simulink model "aerotest"  (R2021b)
settings: Solver=VariableStepAuto  StartTime=0.0  StopTime=10.0  RelTol=1e-3
undefined symbols (not defined in the file or in its folder): admireDB
libraries: simulink_extras x103, simulink x24, aerolibatmos2 x1
(part 7 of 13)

== system aerotest/YawMomentCoefficient/MachRegion2/Cymdna ==
  in_bus : Inport
  Bus Selector : BusSelector  OutputSignals=AeroIn_Bus.dNE,AeroIn_Bus.angleOfAttack_deg,AeroIn_Bus.tflow,AeroIn_Bus.tfhigh,AeroIn_Bus.dNA
  Cymdna_ : Subsystem
  Cymdna : Outport
  wires:
  Bus Selector/2 -> Cymdna_/2(angleOfAttack_deg)  "<angleOfAttack_deg>"
  Bus Selector/1 -> Cymdna_/1(dNE)  "<dNE>"
  Bus Selector/3 -> Cymdna_/3(tflow)  "<tflow>"
  Bus Selector/4 -> Cymdna_/4(tfhigh)  "<tfhigh>"
  Bus Selector/5 -> Cymdna_/5(dNA)  "<dNA>"
  in_bus/1 -> Bus Selector/1  "in_bus"
  Cymdna_/1(Cymdna) -> Cymdna/1

== system aerotest/YawMomentCoefficient/MachRegion2/Cymdr ==
  in_bus : Inport
  Bus Selector : BusSelector  OutputSignals=AeroIn_Bus.angleOfAttack_deg,AeroIn_Bus.rud_deg,AeroIn_Bus.angleOfSideslip_deg,AeroIn_Bus.tflow,AeroIn_Bus.tfhigh,AeroIn_Bus.qacorr,AeroIn_Bus.mach_nd
  Cymdr_ : Subsystem
  Cymdr : Outport
  wires:
  Bus Selector/1 -> Cymdr_/1(angleOfAttack_deg)  "<angleOfAttack_deg>"
  Bus Selector/2 -> Cymdr_/2(dR)  "<rud_deg>"
  Bus Selector/3 -> Cymdr_/3(angleOfSideslip_deg)  "<angleOfSideslip_deg>"
  Bus Selector/4 -> Cymdr_/4(tfhigh)  "<tflow>"
  Bus Selector/5 -> Cymdr_/5(tflow)  "<tfhigh>"
  Bus Selector/6 -> Cymdr_/6(qacorr)  "<qacorr>"
  Bus Selector/7 -> Cymdr_/7(mach_nd)  "<mach_nd>"
  in_bus/1 -> Bus Selector/1  "in_bus"
  Cymdr_/1(Cymdr) -> Cymdr/1

== system aerotest/YawMomentCoefficient/MachRegion2/Cymp ==
  in_bus : Inport
  Bus Selector : BusSelector  OutputSignals=AeroIn_Bus.dN,AeroIn_Bus.angleOfAttack_deg,AeroIn_Bus.tflow,AeroIn_Bus.tfhigh,AeroIn_Bus.pc,AeroIn_Bus.qacorr,AeroIn_Bus.mach_nd
  Cymp_ : Subsystem
  Cymp : Outport
  wires:
  Bus Selector/1 -> Cymp_/1(dN)  "<dN>"
  Bus Selector/2 -> Cymp_/2(angleOfAttack_deg)  "<angleOfAttack_deg>"
  Bus Selector/7 -> Cymp_/7(mach_nd)  "<mach_nd>"
  Bus Selector/3 -> Cymp_/3(tflow)  "<tflow>"
  Bus Selector/6 -> Cymp_/6(qacorr)  "<qacorr>"
  Bus Selector/4 -> Cymp_/4(tfhigh)  "<tfhigh>"
  Bus Selector/5 -> Cymp_/5(pc)  "<pc>"
  in_bus/1 -> Bus Selector/1  "in_bus"
  Cymp_/1(Cymp) -> Cymp/1

== system aerotest/YawMomentCoefficient/MachRegion2/Cympbeta ==
  in_bus : Inport
  Bus Selector : BusSelector  OutputSignals=AeroIn_Bus.angleOfSideslip_deg,AeroIn_Bus.angleOfAttack_deg,AeroIn_Bus.pc,AeroIn_Bus.tflow
  Cympbeta_ : Subsystem
  Cympbeta : Outport
  wires:
  Bus Selector/1 -> Cympbeta_/1(angleOfSideslip_deg)  "<angleOfSideslip_deg>"
  Bus Selector/2 -> Cympbeta_/2(angleOfAttack_deg)  "<angleOfAttack_deg>"
  Bus Selector/3 -> Cympbeta_/3(pc)  "<pc>"
  Bus Selector/4 -> Cympbeta_/4(tflow)  "<tflow>"
  Cympbeta_/1(Cympbeta) -> Cympbeta/1
  in_bus/1 -> Bus Selector/1  "in_bus"

== system aerotest/YawMomentCoefficient/MachRegion2/Cymr ==
  in_bus : Inport
  Bus Selector : BusSelector  OutputSignals=AeroIn_Bus.dN,AeroIn_Bus.angleOfAttack_deg,AeroIn_Bus.tflow,AeroIn_Bus.tfhigh,AeroIn_Bus.rc,AeroIn_Bus.mach_nd,AeroIn_Bus.qacorr
  Cymr_ : Subsystem
  Cymr : Outport
  wires:
  Bus Selector/7 -> Cymr_/7(qacorr)  "<qacorr>"
  Bus Selector/6 -> Cymr_/6(mach_nd)  "<mach_nd>"
  Bus Selector/5 -> Cymr_/5(rc)  "<rc>"
  Bus Selector/4 -> Cymr_/4(tfhigh)  "<tfhigh>"
  Bus Selector/3 -> Cymr_/3(tflow)  "<tflow>"
  Bus Selector/2 -> Cymr_/2(angleOfAttack_deg)  "<angleOfAttack_deg>"
  Bus Selector/1 -> Cymr_/1(dN)  "<dN>"
  in_bus/1 -> Bus Selector/1  "in_bus"
  Cymr_/1(Cymr) -> Cymr/1

== system aerotest/YawMomentCoefficient/MachRegion2/Cymrbeta ==
  in_bus : Inport
  Bus Selector : BusSelector  OutputSignals=AeroIn_Bus.angleOfSideslip_deg,AeroIn_Bus.angleOfAttack_deg,AeroIn_Bus.rc,AeroIn_Bus.tflow
  Cymrbeta_ : Subsystem
  Cymrbeta : Outport
  wires:
  Bus Selector/1 -> Cymrbeta_/1(angleOfSideslip_deg)  "<angleOfSideslip_deg>"
  Bus Selector/2 -> Cymrbeta_/2(angleOfAttack_deg)  "<angleOfAttack_deg>"
  Bus Selector/3 -> Cymrbeta_/3(rc)  "<rc>"
  Bus Selector/4 -> Cymrbeta_/4(tflow)  "<tflow>"
  Cymrbeta_/1(Cymrbeta) -> Cymrbeta/1
  in_bus/1 -> Bus Selector/1  "in_bus"

== system aerotest/YawMomentCoefficient/MachRegion2/eoeff ==
  AeroIn_Bus : Inport
  Bus Selector : BusSelector  OutputSignals=mach_nd
  CYMDAYOD_M : Lookup_n-D  NumberOfTableDimensions=1  BreakpointsForDimension1=admireDB.aerodata_asym_ext.CYMDAYOD.breakpoints.M  BreakpointsForDimension3=[5, 7]  Table=admireDB.aerodata_asym_ext.CYMDAYOD.newTable  ExtrapMethod=Clip  InternalRulePriority=Speed  RndMeth=Simplest  InputSameDT=on
  Constant : Constant
  Sum : Sum  Inputs=-+|
  eoeff : Outport
  eieff : Outport  Port=2
  wires:
  Sum/1 -> eieff/1
  CYMDAYOD_M/1 -> eoeff/1, Sum/1
  Constant/1 -> Sum/2
  Bus Selector/1 -> CYMDAYOD_M/1  "<mach_nd>"
  AeroIn_Bus/1 -> Bus Selector/1

== system aerotest/YawMomentCoefficient/MachRegion3/Cymbasic ==
  Constant : Constant  Value=0
  Cymbasic : Outport
  wires:
  Constant/1 -> Cymbasic/1

== system aerotest/YawMomentCoefficient/MachRegion3/Cymbcai ==
  in_bus : Inport
  Bus Selector : BusSelector  OutputSignals=AeroIn_Bus.cai,AeroIn_Bus.angleOfAttack_deg,AeroIn_Bus.angleOfSideslip_deg
  Cymbcai_ : Subsystem
  Cymbcai : Outport
  wires:
  Bus Selector/3 -> Cymbcai_/3(angleOfSideslip_deg)  "<angleOfSideslip_deg>"
  Bus Selector/2 -> Cymbcai_/2(angleOfAttack_deg)  "<angleOfAttack_deg>"
  Bus Selector/1 -> Cymbcai_/1(CAI)  "<cai>"
  in_bus/1 -> Bus Selector/1  "in_bus"
  Cymbcai_/1(Cymbcai) -> Cymbcai/1

== system aerotest/YawMomentCoefficient/MachRegion3/Cymbde ==
  in_bus : Inport
  Bus Selector : BusSelector  OutputSignals=AeroIn_Bus.angleOfAttack_deg,AeroIn_Bus.dEI,AeroIn_Bus.angleOfSideslip_deg,AeroIn_Bus.dEY,eieff,eoeff,AeroIn_Bus.mach_nd
  Cymbde_ : Subsystem
  Cymbde : Outport
  wires:
  Bus Selector/7 -> Cymbde_/7(mach_nd)  "<mach_nd>"
  Bus Selector/6 -> Cymbde_/6(eoeff)  "<eoeff>"
  Bus Selector/5 -> Cymbde_/5(eieff)  "<eieff>"
  Bus Selector/4 -> Cymbde_/4(dEY)  "<dEY>"
  Bus Selector/3 -> Cymbde_/3(angleOfSideslip_deg)  "<angleOfSideslip_deg>"
  Bus Selector/2 -> Cymbde_/2(dEI)  "<dEI>"
  Bus Selector/1 -> Cymbde_/1(angleOfAttack_deg)  "<angleOfAttack_deg>"
  Cymbde_/1(Cymbde) -> Cymbde/1
  in_bus/1 -> Bus Selector/1  "in_bus"

== system aerotest/YawMomentCoefficient/MachRegion3/Cymbdle ==
  in_bus : Inport
  Bus Selector : BusSelector  OutputSignals=AeroIn_Bus.angleOfAttack_deg,AeroIn_Bus.dEI,AeroIn_Bus.mach_nd,AeroIn_Bus.dEY,eieff,eoeff,AeroIn_Bus.angleOfSideslip_deg,AeroIn_Bus.lef_deg
  Cymbdle_ : Subsystem
  Cymbdle : Outport
  wires:
  Bus Selector/8 -> Cymbdle_/8(dLE)  "<lef_deg>"
  Bus Selector/7 -> Cymbdle_/7(angleOfSideslip_deg)  "<angleOfSideslip_deg>"
  Bus Selector/6 -> Cymbdle_/6(eoeff)  "<eoeff>"
  Bus Selector/5 -> Cymbdle_/5(eieff)  "<eieff>"
  Bus Selector/4 -> Cymbdle_/4(dEY)  "<dEY>"
  Bus Selector/3 -> Cymbdle_/3(mach_nd)  "<mach_nd>"
  Bus Selector/2 -> Cymbdle_/2(dEI)  "<dEI>"
  Bus Selector/1 -> Cymbdle_/1(angleOfAttack_deg)  "<angleOfAttack_deg>"
  Cymbdle_/1(Cymbdle) -> Cymbdle/1
  in_bus/1 -> Bus Selector/1  "in_bus"

== system aerotest/YawMomentCoefficient/MachRegion3/Cymbdn ==
  in_bus : Inport
  Bus Selector : BusSelector  OutputSignals=AeroIn_Bus.angleOfAttack_deg,AeroIn_Bus.dN,AeroIn_Bus.angleOfSideslip_deg
  Cymbdn_ : Subsystem
  Cymbdn : Outport
  wires:
  Bus Selector/1 -> Cymbdn_/1(angleOfAttack_deg)  "<angleOfAttack_deg>"
  Bus Selector/3 -> Cymbdn_/3(angleOfSideslip_deg)  "<angleOfSideslip_deg>"
  Bus Selector/2 -> Cymbdn_/2(dN)  "<dN>"
  in_bus/1 -> Bus Selector/1  "in_bus"
  Cymbdn_/1(Cymbdn) -> Cymbdn/1

== system aerotest/YawMomentCoefficient/MachRegion3/Cymbeta ==
  in_bus : Inport
  Bus Selector : BusSelector  OutputSignals=AeroIn_Bus.angleOfSideslip_deg,AeroIn_Bus.angleOfAttack_deg,AeroIn_Bus.mach_nd,AeroIn_Bus.qacorr
  Cymbeta_ : Subsystem
  Cymbeta : Outport
  wires:
  Bus Selector/1 -> Cymbeta_/1(angleOfSideslip_deg)  "<angleOfSideslip_deg>"
  Bus Selector/2 -> Cymbeta_/2(angleOfAttack_deg)  "<angleOfAttack_deg>"
  Bus Selector/3 -> Cymbeta_/3(mach_nd)  "<mach_nd>"
  Bus Selector/4 -> Cymbeta_/4(qacorr)  "<qacorr>"
  in_bus/1 -> Bus Selector/1  "in_bus"
  Cymbeta_/1(Cymbeta) -> Cymbeta/1

== system aerotest/YawMomentCoefficient/MachRegion3/Cymbetad ==
  in_bus : Inport
  Bus Selector : BusSelector  OutputSignals=AeroIn_Bus.angleOfAttack_deg,AeroIn_Bus.mach_nd,AeroIn_Bus.betad
  Cymbetad_ : Subsystem
  Cymbetad : Outport
  wires:
  Bus Selector/3 -> Cymbetad_/3(betad)  "<betad>"
  Bus Selector/2 -> Cymbetad_/2(mach_nd)  "<mach_nd>"
  Bus Selector/1 -> Cymbetad_/1(angleOfAttack_deg)  "<angleOfAttack_deg>"
  Cymbetad_/1(Cymbetad) -> Cymbetad/1
  in_bus/1 -> Bus Selector/1  "in_bus"

== system aerotest/YawMomentCoefficient/MachRegion3/Cymblg ==
  in_bus : Inport
  Bus Selector : BusSelector  OutputSignals=AeroIn_Bus.angleOfSideslip_deg,AeroIn_Bus.lg_bool,AeroIn_Bus.angleOfAttack_deg
  Cymblg_ : Subsystem
  Cymblg : Outport
  wires:
  Bus Selector/3 -> Cymblg_/3(angleOfAttack_deg)  "<angleOfAttack_deg>"
  Bus Selector/1 -> Cymblg_/1(angleOfSideslip_deg)  "<angleOfSideslip_deg>"
  Bus Selector/2 -> Cymblg_/2(dLG)  "<lg_bool>"
  Cymblg_/1(Cymblg) -> Cymblg/1
  in_bus/1 -> Bus Selector/1  "in_bus"

== system aerotest/YawMomentCoefficient/MachRegion3/Cymdai ==
  in_bus : Inport
  Bus Selector : BusSelector  OutputSignals=AeroIn_Bus.angleOfAttack_deg,AeroIn_Bus.dAI,AeroIn_Bus.mach_nd,AeroIn_Bus.dEI,AeroIn_Bus.qacorr,eieff
  Cymdai_ : Subsystem
  Cymdai : Outport
  wires:
  Bus Selector/6 -> Cymdai_/6(eieff)  "<eieff>"
  Bus Selector/5 -> Cymdai_/5(qacorr)  "<qacorr>"
  Bus Selector/4 -> Cymdai_/4(dEI)  "<dEI>"
  Bus Selector/3 -> Cymdai_/3(mach_nd)  "<mach_nd>"
  Bus Selector/2 -> Cymdai_/2(dAI)  "<dAI>"
  Bus Selector/1 -> Cymdai_/1(angleOfAttack_deg)  "<angleOfAttack_deg>"
  Cymdai_/1(Cymdai) -> Cymdai/1
  in_bus/1 -> Bus Selector/1  "in_bus"

== system aerotest/YawMomentCoefficient/MachRegion3/Cymdaib ==
  Cymdaib_ : Constant  Value=0
  Cymdaib : Outport
  wires:
  Cymdaib_/1 -> Cymdaib/1

== system aerotest/YawMomentCoefficient/MachRegion3/Cymday ==
  in_bus : Inport
  Bus Selector : BusSelector  OutputSignals=AeroIn_Bus.angleOfAttack_deg,AeroIn_Bus.dAY,AeroIn_Bus.mach_nd,AeroIn_Bus.dEY,eoeff,AeroIn_Bus.qacorr
  Cymday_ : Subsystem
  Cymday : Outport
  wires:
  Bus Selector/6 -> Cymday_/6(qacorr)  "<qacorr>"
  Bus Selector/5 -> Cymday_/5(eoef)  "<eoeff>"
  Bus Selector/1 -> Cymday_/1(angleOfAttack_deg)  "<angleOfAttack_deg>"
  Bus Selector/4 -> Cymday_/4(dEY)  "<dEY>"
  Bus Selector/2 -> Cymday_/2(dAY)  "<dAY>"
  Bus Selector/3 -> Cymday_/3(mach_nd)  "<mach_nd>"
  in_bus/1 -> Bus Selector/1  "in_bus"
  Cymday_/1(Cymday) -> Cymday/1

== system aerotest/YawMomentCoefficient/MachRegion3/Cymdayb ==
  Cymdayb_ : Constant  Value=0
  Cymdayb : Outport
  wires:
  Cymdayb_/1 -> Cymdayb/1

== system aerotest/YawMomentCoefficient/MachRegion3/Cymdna ==
  in_bus : Inport
  Bus Selector : BusSelector  OutputSignals=AeroIn_Bus.angleOfAttack_deg,AeroIn_Bus.mach_nd,AeroIn_Bus.dNA
  Cymdna_ : Subsystem
  Cymdna : Outport
  wires:
  Bus Selector/1 -> Cymdna_/1(angleOfAttack_deg)  "<angleOfAttack_deg>"
  Bus Selector/2 -> Cymdna_/2(mach_nd)  "<mach_nd>"
  Bus Selector/3 -> Cymdna_/3(dNA)  "<dNA>"
  in_bus/1 -> Bus Selector/1  "in_bus"
  Cymdna_/1(Cymdna) -> Cymdna/1

== system aerotest/YawMomentCoefficient/MachRegion3/Cymdr ==
  in_bus : Inport
  Bus Selector : BusSelector  OutputSignals=AeroIn_Bus.angleOfAttack_deg,AeroIn_Bus.mach_nd,AeroIn_Bus.rud_deg,AeroIn_Bus.qacorr
  Cymdr_ : Subsystem
  Cymdr : Outport
  wires:
  Bus Selector/1 -> Cymdr_/1(angleOfAttack_deg)  "<angleOfAttack_deg>"
  Bus Selector/2 -> Cymdr_/2(mach_nd)  "<mach_nd>"
  Bus Selector/3 -> Cymdr_/3(dR)  "<rud_deg>"
  Bus Selector/4 -> Cymdr_/4(qacorr)  "<qacorr>"
  in_bus/1 -> Bus Selector/1  "in_bus"
  Cymdr_/1(Cymdr) -> Cymdr/1

== system aerotest/YawMomentCoefficient/MachRegion3/Cymp ==
  in_bus : Inport
  Bus Selector : BusSelector  OutputSignals=AeroIn_Bus.angleOfAttack_deg,AeroIn_Bus.mach_nd,AeroIn_Bus.qacorr,AeroIn_Bus.pc
  Cymp_ : Subsystem
  Cymp : Outport
  wires:
  Bus Selector/1 -> Cymp_/1(angleOfAttack_deg)  "<angleOfAttack_deg>"
  Bus Selector/2 -> Cymp_/2(mach_nd)  "<mach_nd>"
  Bus Selector/3 -> Cymp_/3(qacorr)  "<qacorr>"
  Bus Selector/4 -> Cymp_/4(pc)  "<pc>"
  in_bus/1 -> Bus Selector/1  "in_bus"
  Cymp_/1(Cymp) -> Cymp/1

== system aerotest/YawMomentCoefficient/MachRegion3/Cympbeta ==
  Cympbeta_ : Constant  Value=0
  Cympbeta : Outport
  wires:
  Cympbeta_/1 -> Cympbeta/1

== system aerotest/YawMomentCoefficient/MachRegion3/Cymr ==
  in_bus : Inport
  Bus Selector : BusSelector  OutputSignals=AeroIn_Bus.mach_nd,AeroIn_Bus.angleOfAttack_deg,AeroIn_Bus.dN,AeroIn_Bus.qacorr,AeroIn_Bus.rc
  Cymr_ : Subsystem
  Cymr : Outport
  wires:
  Bus Selector/1 -> Cymr_/1(mach_nd)  "<mach_nd>"
  Bus Selector/2 -> Cymr_/2(angleOfAttack_deg)  "<angleOfAttack_deg>"
  Bus Selector/3 -> Cymr_/3(dN)  "<dN>"
  Bus Selector/4 -> Cymr_/4(qacorr)  "<qacorr>"
  Bus Selector/5 -> Cymr_/5(rc)  "<rc>"
  in_bus/1 -> Bus Selector/1  "in_bus"
  Cymr_/1(Cymr) -> Cymr/1

== system aerotest/YawMomentCoefficient/MachRegion3/Cymrbeta ==
  Cymrbeta_ : Constant  Value=0
  Cymrbeta : Outport
  wires:
  Cymrbeta_/1 -> Cymrbeta/1

== system aerotest/YawMomentCoefficient/MachRegion3/eoeff ==
  AeroIn_Bus : Inport
  Bus Selector : BusSelector  OutputSignals=mach_nd
  CYMDAYOD_M : Lookup_n-D  NumberOfTableDimensions=1  BreakpointsForDimension1=admireDB.aerodata_asym_ext.CYMDAYOD.breakpoints.M  BreakpointsForDimension3=[5, 7]  Table=admireDB.aerodata_asym_ext.CYMDAYOD.newTable  ExtrapMethod=Clip  InternalRulePriority=Speed  RndMeth=Simplest  InputSameDT=on
  Constant : Constant
  Sum : Sum  Inputs=-+|
  eoeff : Outport
  eieff : Outport  Port=2
  wires:
  Sum/1 -> eieff/1
  CYMDAYOD_M/1 -> eoeff/1, Sum/1
  Constant/1 -> Sum/2
  Bus Selector/1 -> CYMDAYOD_M/1  "<mach_nd>"
  AeroIn_Bus/1 -> Bus Selector/1

== system aerotest/YawMomentCoefficient/MachRegion4/Cymbasic ==
  Constant : Constant  Value=0
  Cymbasic : Outport
  wires:
  Constant/1 -> Cymbasic/1

== system aerotest/YawMomentCoefficient/MachRegion4/Cymbcai ==
  in_bus : Inport
  Bus Selector : BusSelector  OutputSignals=AeroIn_Bus.cai,AeroIn_Bus.angleOfAttack_deg,AeroIn_Bus.angleOfSideslip_deg
  Cymbcai_ : Subsystem
  Cymbcai : Outport
  wires:
  Cymbcai_/1(Cymbcai) -> Cymbcai/1
  in_bus/1 -> Bus Selector/1  "in_bus"
  Bus Selector/1 -> Cymbcai_/1(CAI)  "<cai>"
  Bus Selector/2 -> Cymbcai_/2(angleOfAttack_deg)  "<angleOfAttack_deg>"
  Bus Selector/3 -> Cymbcai_/3(angleOfSideslip_deg)  "<angleOfSideslip_deg>"

== system aerotest/YawMomentCoefficient/MachRegion4/Cymbde ==
  in_bus : Inport
  Bus Selector : BusSelector  OutputSignals=AeroIn_Bus.angleOfAttack_deg,AeroIn_Bus.dEI,AeroIn_Bus.angleOfSideslip_deg,AeroIn_Bus.dEY,eieff,eoeff,AeroIn_Bus.mach_nd
  Cymbde_ : Subsystem
  Cymbde : Outport
  wires:
  in_bus/1 -> Bus Selector/1  "in_bus"
  Cymbde_/1(Cymbde) -> Cymbde/1
  Bus Selector/1 -> Cymbde_/1(angleOfAttack_deg)  "<angleOfAttack_deg>"
  Bus Selector/2 -> Cymbde_/2(dEI)  "<dEI>"
  Bus Selector/3 -> Cymbde_/3(angleOfSideslip_deg)  "<angleOfSideslip_deg>"
  Bus Selector/4 -> Cymbde_/4(dEY)  "<dEY>"
  Bus Selector/5 -> Cymbde_/5(eieff)  "<eieff>"
  Bus Selector/6 -> Cymbde_/6(eoeff)  "<eoeff>"
  Bus Selector/7 -> Cymbde_/7(mach_nd)  "<mach_nd>"

== system aerotest/YawMomentCoefficient/MachRegion4/Cymbdle ==
  in_bus : Inport
  Bus Selector : BusSelector  OutputSignals=AeroIn_Bus.angleOfAttack_deg,AeroIn_Bus.dEI,AeroIn_Bus.mach_nd,AeroIn_Bus.dEY,eieff,eoeff,AeroIn_Bus.angleOfSideslip_deg,AeroIn_Bus.lef_deg
  Cymbdle_ : Subsystem
  Cymbdle : Outport
  wires:
  in_bus/1 -> Bus Selector/1  "in_bus"
  Cymbdle_/1(Cymbdle) -> Cymbdle/1
  Bus Selector/1 -> Cymbdle_/1(angleOfAttack_deg)  "<angleOfAttack_deg>"
  Bus Selector/2 -> Cymbdle_/2(dEI)  "<dEI>"
  Bus Selector/3 -> Cymbdle_/3(mach_nd)  "<mach_nd>"
  Bus Selector/4 -> Cymbdle_/4(dEY)  "<dEY>"
  Bus Selector/5 -> Cymbdle_/5(eieff)  "<eieff>"
  Bus Selector/6 -> Cymbdle_/6(eoeff)  "<eoeff>"
  Bus Selector/7 -> Cymbdle_/7(angleOfSideslip_deg)  "<angleOfSideslip_deg>"
  Bus Selector/8 -> Cymbdle_/8(dLE)  "<lef_deg>"

== system aerotest/YawMomentCoefficient/MachRegion4/Cymbdn ==
  in_bus : Inport
  Bus Selector : BusSelector  OutputSignals=AeroIn_Bus.angleOfAttack_deg,AeroIn_Bus.dN,AeroIn_Bus.angleOfSideslip_deg
  Cymbdn_ : Subsystem
  Cymbdn : Outport
  wires:
  Cymbdn_/1(Cymbdn) -> Cymbdn/1
  in_bus/1 -> Bus Selector/1  "in_bus"
  Bus Selector/2 -> Cymbdn_/2(dN)  "<dN>"
  Bus Selector/3 -> Cymbdn_/3(angleOfSideslip_deg)  "<angleOfSideslip_deg>"
  Bus Selector/1 -> Cymbdn_/1(angleOfAttack_deg)  "<angleOfAttack_deg>"

== system aerotest/YawMomentCoefficient/MachRegion4/Cymbeta ==
  in_bus : Inport
  Bus Selector : BusSelector  OutputSignals=AeroIn_Bus.angleOfSideslip_deg,AeroIn_Bus.angleOfAttack_deg,AeroIn_Bus.mach_nd,AeroIn_Bus.qacorr
  Cymbeta_ : Subsystem
  Cymbeta : Outport
  wires:
  Cymbeta_/1(Cymbeta) -> Cymbeta/1
  in_bus/1 -> Bus Selector/1  "in_bus"
  Bus Selector/4 -> Cymbeta_/4(qacorr)  "<qacorr>"
  Bus Selector/3 -> Cymbeta_/3(mach_nd)  "<mach_nd>"
  Bus Selector/2 -> Cymbeta_/2(angleOfAttack_deg)  "<angleOfAttack_deg>"
  Bus Selector/1 -> Cymbeta_/1(angleOfSideslip_deg)  "<angleOfSideslip_deg>"

== system aerotest/YawMomentCoefficient/MachRegion4/Cymbetad ==
  in_bus : Inport
  Bus Selector : BusSelector  OutputSignals=AeroIn_Bus.angleOfAttack_deg,AeroIn_Bus.mach_nd,AeroIn_Bus.betad
  Cymbetad_ : Subsystem
  Cymbetad : Outport
  wires:
  in_bus/1 -> Bus Selector/1  "in_bus"
  Cymbetad_/1(Cymbetad) -> Cymbetad/1
  Bus Selector/1 -> Cymbetad_/1(angleOfAttack_deg)  "<angleOfAttack_deg>"
  Bus Selector/2 -> Cymbetad_/2(mach_nd)  "<mach_nd>"
  Bus Selector/3 -> Cymbetad_/3(betad)  "<betad>"

== system aerotest/YawMomentCoefficient/MachRegion4/Cymblg ==
  in_bus : Inport
  Bus Selector : BusSelector  OutputSignals=AeroIn_Bus.angleOfSideslip_deg,AeroIn_Bus.lg_bool,AeroIn_Bus.angleOfAttack_deg
  Cymblg_ : Subsystem
  Cymblg : Outport
  wires:
  in_bus/1 -> Bus Selector/1  "in_bus"
  Cymblg_/1(Cymblg) -> Cymblg/1
  Bus Selector/2 -> Cymblg_/2(dLG)  "<lg_bool>"
  Bus Selector/1 -> Cymblg_/1(angleOfSideslip_deg)  "<angleOfSideslip_deg>"
  Bus Selector/3 -> Cymblg_/3(angleOfAttack_deg)  "<angleOfAttack_deg>"

== system aerotest/YawMomentCoefficient/MachRegion4/Cymdai ==
  in_bus : Inport
  Bus Selector : BusSelector  OutputSignals=AeroIn_Bus.dAI,AeroIn_Bus.angleOfAttack_deg,AeroIn_Bus.dEI,AeroIn_Bus.mach_nd,eieff,AeroIn_Bus.qacorr
  Cymdai_ : Subsystem
  Cymdai : Outport
  wires:
  Bus Selector/1 -> Cymdai_/1(dAI)  "<dAI>"
  Bus Selector/2 -> Cymdai_/2(angleOfAttack_deg)  "<angleOfAttack_deg>"
  Bus Selector/3 -> Cymdai_/3(dEI)  "<dEI>"
  Bus Selector/4 -> Cymdai_/4(mach_nd)  "<mach_nd>"
  Bus Selector/5 -> Cymdai_/5(eieff)  "<eieff>"
  Bus Selector/6 -> Cymdai_/6(qacorr)  "<qacorr>"
  in_bus/1 -> Bus Selector/1  "in_bus"
  Cymdai_/1(Cymdai) -> Cymdai/1

== system aerotest/YawMomentCoefficient/MachRegion4/Cymdaib ==
  Cymdaib_ : Constant  Value=0
  Cymdaib : Outport
  wires:
  Cymdaib_/1 -> Cymdaib/1

== system aerotest/YawMomentCoefficient/MachRegion4/Cymday ==
  in_bus : Inport
  Bus Selector : BusSelector  OutputSignals=AeroIn_Bus.angleOfAttack_deg,AeroIn_Bus.dEY,AeroIn_Bus.mach_nd,AeroIn_Bus.qacorr,eoeff,AeroIn_Bus.dAY
  Cymday_ : Subsystem
  Cymday : Outport
  wires:
  Bus Selector/6 -> Cymday_/6(dAY)  "<dAY>"
  Bus Selector/5 -> Cymday_/5(eoeff)  "<eoeff>"
  Bus Selector/4 -> Cymday_/4(qacorr)  "<qacorr>"
  Bus Selector/3 -> Cymday_/3(mach_nd)  "<mach_nd>"
  Bus Selector/2 -> Cymday_/2(dEY)  "<dEY>"
  Bus Selector/1 -> Cymday_/1(angleOfAttack_deg)  "<angleOfAttack_deg>"
  Cymday_/1(Cymday) -> Cymday/1
  in_bus/1 -> Bus Selector/1  "in_bus"

== system aerotest/YawMomentCoefficient/MachRegion4/Cymdayb ==
  Cymdayb_ : Constant  Value=0
  Cymdayb : Outport
  wires:
  Cymdayb_/1 -> Cymdayb/1

== system aerotest/YawMomentCoefficient/MachRegion4/Cymdna ==
  in_bus : Inport
  Bus Selector : BusSelector  OutputSignals=AeroIn_Bus.angleOfAttack_deg,AeroIn_Bus.mach_nd,AeroIn_Bus.dNA
  Cymdna_ : Subsystem
  Cymdna : Outport
  wires:
  Cymdna_/1(Cymdna) -> Cymdna/1
  in_bus/1 -> Bus Selector/1  "in_bus"
  Bus Selector/3 -> Cymdna_/3(dNA)  "<dNA>"
  Bus Selector/2 -> Cymdna_/2(mach_nd)  "<mach_nd>"
  Bus Selector/1 -> Cymdna_/1(angleOfAttack_deg)  "<angleOfAttack_deg>"

== system aerotest/YawMomentCoefficient/MachRegion4/Cymdr ==
  in_bus : Inport
  Bus Selector : BusSelector  OutputSignals=AeroIn_Bus.angleOfAttack_deg,AeroIn_Bus.mach_nd,AeroIn_Bus.rud_deg,AeroIn_Bus.qacorr
  Cymdr_ : Subsystem
  Cymdr : Outport
  wires:
  Cymdr_/1(Cymdr) -> Cymdr/1
  in_bus/1 -> Bus Selector/1  "in_bus"
  Bus Selector/4 -> Cymdr_/4(qacorr)  "<qacorr>"
  Bus Selector/3 -> Cymdr_/3(dR)  "<rud_deg>"
  Bus Selector/2 -> Cymdr_/2(mach_nd)  "<mach_nd>"
  Bus Selector/1 -> Cymdr_/1(angleOfAttack_deg)  "<angleOfAttack_deg>"

== system aerotest/YawMomentCoefficient/MachRegion4/Cymp ==
  in_bus : Inport
  Bus Selector : BusSelector  OutputSignals=AeroIn_Bus.angleOfAttack_deg,AeroIn_Bus.mach_nd,AeroIn_Bus.qacorr,AeroIn_Bus.pc
  Cymp_ : Subsystem
  Cymp : Outport
  wires:
  Cymp_/1(Cymp) -> Cymp/1
  in_bus/1 -> Bus Selector/1  "in_bus"
  Bus Selector/4 -> Cymp_/4(pc)  "<pc>"
  Bus Selector/3 -> Cymp_/3(qacorr)  "<qacorr>"
  Bus Selector/2 -> Cymp_/2(mach_nd)  "<mach_nd>"
  Bus Selector/1 -> Cymp_/1(angleOfAttack_deg)  "<angleOfAttack_deg>"

== system aerotest/YawMomentCoefficient/MachRegion4/Cympbeta ==
  Cympbeta_ : Constant  Value=0
  Cympbeta : Outport
  wires:
  Cympbeta_/1 -> Cympbeta/1

== system aerotest/YawMomentCoefficient/MachRegion4/Cymr ==
  in_bus : Inport
  Bus Selector : BusSelector  OutputSignals=AeroIn_Bus.mach_nd,AeroIn_Bus.angleOfAttack_deg,AeroIn_Bus.dN,AeroIn_Bus.qacorr,AeroIn_Bus.rc
  Cymr_ : Subsystem
  Cymr : Outport
  wires:
  Cymr_/1(Cymr) -> Cymr/1
  in_bus/1 -> Bus Selector/1  "in_bus"
  Bus Selector/5 -> Cymr_/5(rc)  "<rc>"
  Bus Selector/4 -> Cymr_/4(qacorr)  "<qacorr>"
  Bus Selector/3 -> Cymr_/3(dN)  "<dN>"
  Bus Selector/2 -> Cymr_/2(angleOfAttack_deg)  "<angleOfAttack_deg>"
  Bus Selector/1 -> Cymr_/1(mach_nd)  "<mach_nd>"

== system aerotest/YawMomentCoefficient/MachRegion4/Cymrbeta ==
  Cymrbeta_ : Constant  Value=0
  Cymrbeta : Outport
  wires:
  Cymrbeta_/1 -> Cymrbeta/1

== system aerotest/YawMomentCoefficient/MachRegion4/eoeff ==
  AeroIn_Bus : Inport
  Bus Selector : BusSelector  OutputSignals=mach_nd
  CYMDAYOD_M : Lookup_n-D  NumberOfTableDimensions=1  BreakpointsForDimension1=admireDB.aerodata_asym_ext.CYMDAYOD.breakpoints.M  BreakpointsForDimension3=[5, 7]  Table=admireDB.aerodata_asym_ext.CYMDAYOD.newTable  ExtrapMethod=Clip  InternalRulePriority=Speed  RndMeth=Simplest  InputSameDT=on
  Constant : Constant
  Sum : Sum  Inputs=-+|
  eoeff : Outport
  eieff : Outport  Port=2
  wires:
  AeroIn_Bus/1 -> Bus Selector/1
  Bus Selector/1 -> CYMDAYOD_M/1  "<mach_nd>"
  Constant/1 -> Sum/2
  CYMDAYOD_M/1 -> Sum/1, eoeff/1
  Sum/1 -> eieff/1

== system aerotest/CentripetalForceCoefficient/MachRegion1/Ccbcai/Ccbcai_ ==
  CAI : Inport
  angleOfAttack_deg : Inport  Port=2
  angleOfSideslip_deg : Inport  Port=3
  CCBCAI_CAI_ALFA : Lookup_n-D  BreakpointsForDimension1=admireDB.aerodata_asym_ext.CCBCAI.breakpoints.ALFA  BreakpointsForDimension2=admireDB.aerodata_asym_ext.CCBCAI.breakpoints.CAI  BreakpointsForDimension3=[5, 7]  Table=admireDB.aerodata_asym_ext.CCBCAI.newTable  ExtrapMethod=Clip  InternalRulePriority=Speed  RndMeth=Simplest  InputSameDT=on
      settings: InputPortMap=u0,u1
  Degrees to Radians : simulink_extras/Transformations/Degrees to Radians
  Product : Product  Inputs=**
  Ccbcai : Outport
  wires:
  Degrees to Radians/1 -> Product/2
  angleOfSideslip_deg/1 -> Degrees to Radians/1
  Product/1 -> Ccbcai/1
  CCBCAI_CAI_ALFA/1 -> Product/1
  CAI/1 -> CCBCAI_CAI_ALFA/2
  angleOfAttack_deg/1 -> CCBCAI_CAI_ALFA/1

== system aerotest/CentripetalForceCoefficient/MachRegion1/Ccbde/Ccbde_ ==
  angleOfSideslip_deg : Inport
  dEI : Inport  Port=2
  angleOfAttack_deg : Inport  Port=3
  eieff : Inport  Port=4
  dEY : Inport  Port=5
  eoeff : Inport  Port=6
  Abs : Abs
  CCDEB_ALFA_DE_BETA : Lookup_n-D  NumberOfTableDimensions=3  BreakpointsForDimension1=admireDB.aerodata_asym_ext.CCDEB.breakpoints.ALFA  BreakpointsForDimension2=admireDB.aerodata_asym_ext.CCDEB.breakpoints.DE  BreakpointsForDimension3=admireDB.aerodata_asym_ext.CCDEB.breakpoints.BETA  Table=admireDB.aerodata_asym_ext.CCDEB.newTable  ExtrapMethod=Clip  InternalRulePriority=Speed  RndMeth=Simplest  InputSameDT=on
      settings: InputPortMap=u0,u1,u2
  CCDEB_ALFA_DE_BETA1 : Lookup_n-D  NumberOfTableDimensions=3  BreakpointsForDimension1=admireDB.aerodata_asym_ext.CCDEB.breakpoints.ALFA  BreakpointsForDimension2=admireDB.aerodata_asym_ext.CCDEB.breakpoints.DE  BreakpointsForDimension3=admireDB.aerodata_asym_ext.CCDEB.breakpoints.BETA  Table=admireDB.aerodata_asym_ext.CCDEB.newTable  ExtrapMethod=Clip  InternalRulePriority=Speed  RndMeth=Simplest  InputSameDT=on
      settings: InputPortMap=u0,u1,u2
  Product : Product  Inputs=**
  Product1 : Product  Inputs=**
  Product2 : Product  Inputs=**
  Sign : Signum
  Sum : Sum  Inputs=|++
  Ccbde : Outport
  wires:
  Abs/1 -> CCDEB_ALFA_DE_BETA1/3, CCDEB_ALFA_DE_BETA/3
  angleOfSideslip_deg/1 -> Sign/1, Abs/1
  Product2/1 -> Ccbde/1
  Sign/1 -> Product2/1
  Sum/1 -> Product2/2
  Product1/1 -> Sum/2
  Product/1 -> Sum/1
  CCDEB_ALFA_DE_BETA1/1 -> Product1/1
  eoeff/1 -> Product1/2
  dEY/1 -> CCDEB_ALFA_DE_BETA1/2
  CCDEB_ALFA_DE_BETA/1 -> Product/1
  eieff/1 -> Product/2
  dEI/1 -> CCDEB_ALFA_DE_BETA/2
  angleOfAttack_deg/1 -> CCDEB_ALFA_DE_BETA1/1, CCDEB_ALFA_DE_BETA/1

== system aerotest/CentripetalForceCoefficient/MachRegion1/Ccbdle/Ccbdle_ ==
  dLE : Inport
  angleOfSideslip_deg : Inport  Port=2
  angleOfAttack_deg : Inport  Port=3
  Abs : Abs
  CCDLEB_ALFA_BETA_DLE : Lookup_n-D  NumberOfTableDimensions=3  BreakpointsForDimension1=admireDB.aerodata_asym_ext.CCDLEB.breakpoints.ALFA  BreakpointsForDimension2=admireDB.aerodata_asym_ext.CCDLEB.breakpoints.BETA  BreakpointsForDimension3=admireDB.aerodata_asym_ext.CCDLEB.breakpoints.DLE  Table=admireDB.aerodata_asym_ext.CCDLEB.newTable  ExtrapMethod=Clip  InternalRulePriority=Speed  RndMeth=Simplest  InputSameDT=on
      settings: InputPortMap=u0,u1,u2
  Product : Product  Inputs=**
  Sign : Signum
  Ccbdle : Outport
  wires:
  Product/1 -> Ccbdle/1
  Sign/1 -> Product/2
  CCDLEB_ALFA_BETA_DLE/1 -> Product/1
  Abs/1 -> CCDLEB_ALFA_BETA_DLE/2
  angleOfAttack_deg/1 -> CCDLEB_ALFA_BETA_DLE/1
  angleOfSideslip_deg/1 -> Sign/1, Abs/1
  dLE/1 -> CCDLEB_ALFA_BETA_DLE/3

== system aerotest/CentripetalForceCoefficient/MachRegion1/Ccbdn/Ccbdn_ ==
  angleOfSideslip_deg : Inport
  dN : Inport  Port=2
  angleOfAttack_deg : Inport  Port=3
  Abs : Abs
  CCDNB_ALFA_DN_BETA : Lookup_n-D  NumberOfTableDimensions=3  BreakpointsForDimension1=admireDB.aerodata_asym_ext.CCDNB.breakpoints.ALFA  BreakpointsForDimension2=admireDB.aerodata_asym_ext.CCDNB.breakpoints.DN  BreakpointsForDimension3=admireDB.aerodata_asym_ext.CCDNB.breakpoints.BETA  Table=admireDB.aerodata_asym_ext.CCDNB.newTable  ExtrapMethod=Clip  InternalRulePriority=Speed  RndMeth=Simplest  InputSameDT=on
      settings: InputPortMap=u0,u1,u2
  Product : Product  Inputs=**
  Sign : Signum
  Ccbdn : Outport
  wires:
  Abs/1 -> CCDNB_ALFA_DN_BETA/3
  angleOfAttack_deg/1 -> CCDNB_ALFA_DN_BETA/1
  Product/1 -> Ccbdn/1
  Sign/1 -> Product/2
  CCDNB_ALFA_DN_BETA/1 -> Product/1
  dN/1 -> CCDNB_ALFA_DN_BETA/2
  angleOfSideslip_deg/1 -> Abs/1, Sign/1

== system aerotest/CentripetalForceCoefficient/MachRegion1/Ccbeta/Ccbeta_ ==
  angleOfSideslip_deg : Inport
  angleOfAttack_deg : Inport  Port=2
  qacorr : Inport  Port=3
  mach_nd : Inport  Port=4
  Abs : Abs
  CCBAL_BETA_ALFA : Lookup_n-D  BreakpointsForDimension1=admireDB.aerodata_asym_ext.CCBAL.breakpoints.ALFA  BreakpointsForDimension2=admireDB.aerodata_asym_ext.CCBAL.breakpoints.BETA  BreakpointsForDimension3=[5, 7]  Table=admireDB.aerodata_asym_ext.CCBAL.newTable  ExtrapMethod=Clip  InternalRulePriority=Speed  RndMeth=Simplest  InputSameDT=on
      settings: InputPortMap=u0,u1
  CCEB_QA_M : Lookup_n-D  BreakpointsForDimension1=admireDB.aerodata_asym_ext.CCEB.breakpoints.M  BreakpointsForDimension2=admireDB.aerodata_asym_ext.CCEB.breakpoints.QA  BreakpointsForDimension3=[5, 7]  Table=admireDB.aerodata_asym_ext.CCEB.newTable  ExtrapMethod=Clip  InternalRulePriority=Speed  RndMeth=Simplest  InputSameDT=on
      settings: InputPortMap=u0,u1
  Product : Product  Inputs=***
  Sign : Signum
  Ccbeta : Outport
  wires:
  Product/1 -> Ccbeta/1
  Sign/1 -> Product/1
  CCBAL_BETA_ALFA/1 -> Product/2
  CCEB_QA_M/1 -> Product/3
  Abs/1 -> CCBAL_BETA_ALFA/2
  angleOfSideslip_deg/1 -> Abs/1, Sign/1
  angleOfAttack_deg/1 -> CCBAL_BETA_ALFA/1
  qacorr/1 -> CCEB_QA_M/2
  mach_nd/1 -> CCEB_QA_M/1

== system aerotest/CentripetalForceCoefficient/MachRegion1/Ccbetad/Ccbetad_ ==
  angleOfAttack_deg : Inport
  betad : Inport  Port=2
  CCBDL_ALFA : Lookup_n-D  NumberOfTableDimensions=1  BreakpointsForDimension1=admireDB.aerodata_asym_ext.CCBDL.breakpoints.ALFA  BreakpointsForDimension3=[5, 7]  Table=admireDB.aerodata_asym_ext.CCBDL.newTable  ExtrapMethod=Clip  InternalRulePriority=Speed  RndMeth=Simplest  InputSameDT=on
  Product : Product
  Ccbetad : Outport
  wires:
  Product/1 -> Ccbetad/1
  betad/1 -> Product/2
  CCBDL_ALFA/1 -> Product/1
  angleOfAttack_deg/1 -> CCBDL_ALFA/1

== system aerotest/CentripetalForceCoefficient/MachRegion1/Ccblg/Ccblg_ ==
  dLG : Inport
  angleOfAttack_deg : Inport  Port=2
  angleOfSideslip_deg : Inport  Port=3
  CCBLST_NG_DOOR_ALFA : Lookup_n-D  BreakpointsForDimension1=admireDB.aerodata_asym_ext.CCBLST.breakpoints.ALFA  BreakpointsForDimension2=admireDB.aerodata_asym_ext.CCBLST.breakpoints.NG_DOOR  BreakpointsForDimension3=[5, 7]  Table=admireDB.aerodata_asym_ext.CCBLST.newTable  ExtrapMethod=Clip  InternalRulePriority=Speed  RndMeth=Simplest  InputSameDT=on
      settings: InputPortMap=u0,u1
  Degrees to Radians : simulink_extras/Transformations/Degrees to Radians
  Product : Product  Inputs=***
  Ccblg : Outport
  wires:
  Product/1 -> Ccblg/1
  Degrees to Radians/1 -> Product/2
  angleOfSideslip_deg/1 -> Degrees to Radians/1
  CCBLST_NG_DOOR_ALFA/1 -> Product/1
  dLG/1 -> Product/3, CCBLST_NG_DOOR_ALFA/2
  angleOfAttack_deg/1 -> CCBLST_NG_DOOR_ALFA/1

== system aerotest/CentripetalForceCoefficient/MachRegion1/Ccdai/Ccdai_ ==
  dAI : Inport
  angleOfAttack_deg : Inport  Port=2
  dEI : Inport  Port=3
  eieff : Inport  Port=4
  qacorr : Inport  Port=5
  mach_nd : Inport  Port=6
  Abs : Abs
  CCDAAL_DA_ALFA : Lookup_n-D  BreakpointsForDimension1=admireDB.aerodata_asym_ext.CCDAAL.breakpoints.ALFA  BreakpointsForDimension2=admireDB.aerodata_asym_ext.CCDAAL.breakpoints.DA  BreakpointsForDimension3=[5, 7]  Table=admireDB.aerodata_asym_ext.CCDAAL.newTable  ExtrapMethod=Clip  InternalRulePriority=Speed  RndMeth=Simplest  InputSameDT=on
      settings: InputPortMap=u0,u1
  CCDAL_DE_ALFA : Lookup_n-D  BreakpointsForDimension1=admireDB.aerodata_asym_ext.CCDAL.breakpoints.ALFA  BreakpointsForDimension2=admireDB.aerodata_asym_ext.CCDAL.breakpoints.DE  BreakpointsForDimension3=[5, 7]  Table=admireDB.aerodata_asym_ext.CCDAL.newTable  ExtrapMethod=Clip  InternalRulePriority=Speed  RndMeth=Simplest  InputSameDT=on
      settings: InputPortMap=u0,u1
  CCDAL_DE_ALFA_1 : Lookup_n-D  BreakpointsForDimension1=admireDB.aerodata_asym_ext.CCDAL.breakpoints.ALFA  BreakpointsForDimension2=admireDB.aerodata_asym_ext.CCDAL.breakpoints.DE  BreakpointsForDimension3=[5, 7]  Table=admireDB.aerodata_asym_ext.CCDAL.newTable  ExtrapMethod=Clip  InternalRulePriority=Speed  RndMeth=Simplest  InputSameDT=on
      settings: InputPortMap=u0,u1
  CCEDAI_QA_M : Lookup_n-D  BreakpointsForDimension1=admireDB.aerodata_asym_ext.CCEDAI.breakpoints.M  BreakpointsForDimension2=admireDB.aerodata_asym_ext.CCEDAI.breakpoints.QA  BreakpointsForDimension3=[5, 7]  Table=admireDB.aerodata_asym_ext.CCEDAI.newTable  ExtrapMethod=Clip  InternalRulePriority=Speed  RndMeth=Simplest  InputSameDT=on
      settings: InputPortMap=u0,u1
  Degrees to Radians : simulink_extras/Transformations/Degrees to Radians
  Product : Product  Inputs=**
  Product1 : Product  Inputs=**
  Product2 : Product  Inputs=3
  Sign : Signum
  Sum : Sum  Inputs=|++
  Sum1 : Sum  Inputs=|+-
  dE_cnst : Constant  Value=0.0
  Ccdai : Outport
  wires:
  Sum1/1 -> Product1/2
  Product2/1 -> Ccdai/1
  CCEDAI_QA_M/1 -> Product2/3
  qacorr/1 -> CCEDAI_QA_M/2
  mach_nd/1 -> CCEDAI_QA_M/1
  Sum/1 -> Product2/1
  eieff/1 -> Product2/2
  Product1/1 -> Sum/2
  Degrees to Radians/1 -> Product1/1
  CCDAL_DE_ALFA_1/1 -> Sum1/2
  CCDAL_DE_ALFA/1 -> Sum1/1
  angleOfAttack_deg/1 -> CCDAL_DE_ALFA/1, CCDAL_DE_ALFA_1/1, CCDAAL_DA_ALFA/1
  dEI/1 -> CCDAL_DE_ALFA/2
  dE_cnst/1 -> CCDAL_DE_ALFA_1/2
  Product/1 -> Sum/1
  Abs/1 -> CCDAAL_DA_ALFA/2
  Sign/1 -> Product/1
  CCDAAL_DA_ALFA/1 -> Product/2
  dAI/1 -> Sign/1, Abs/1, Degrees to Radians/1

== system aerotest/CentripetalForceCoefficient/MachRegion1/Ccdaib/Ccdaib_ ==
  angleOfAttack_deg : Inport
  dAI : Inport  Port=2
  angleOfSideslip_deg : Inport  Port=3
  eieff : Inport  Port=4
  Abs : Abs
  Abs1 : Abs
  Abs2 : Abs
  CCDABAL_ALFA : Lookup_n-D  NumberOfTableDimensions=1  BreakpointsForDimension1=admireDB.aerodata_asym_ext.CCDABAL.breakpoints.ALFA  BreakpointsForDimension3=[5, 7]  Table=admireDB.aerodata_asym_ext.CCDABAL.newTable  ExtrapMethod=Clip  InternalRulePriority=Speed  RndMeth=Simplest  InputSameDT=on
  Constant : Constant  Value=30
  Constant1 : Constant  Value=20
  Product : Product  Inputs=**/*/*
  Ccdaib : Outport
  wires:
  Abs2/1 -> CCDABAL_ALFA/1
  Constant1/1 -> Product/5
  Abs1/1 -> Product/4
  angleOfSideslip_deg/1 -> Abs1/1
  Constant/1 -> Product/3
  Abs/1 -> Product/2
  CCDABAL_ALFA/1 -> Product/1
  Product/1 -> Ccdaib/1
  angleOfAttack_deg/1 -> Abs2/1
  dAI/1 -> Abs/1
  eieff/1 -> Product/6

== system aerotest/CentripetalForceCoefficient/MachRegion1/Ccday/Ccday_ ==
  dAY : Inport
  angleOfAttack_deg : Inport  Port=2
  dEY : Inport  Port=3
  eoeff : Inport  Port=4
  qacorr : Inport  Port=5
  mach_nd : Inport  Port=6
  Abs : Abs
  CCDAAL_DA_ALFA : Lookup_n-D  BreakpointsForDimension1=admireDB.aerodata_asym_ext.CCDAAL.breakpoints.ALFA  BreakpointsForDimension2=admireDB.aerodata_asym_ext.CCDAAL.breakpoints.DA  BreakpointsForDimension3=[5, 7]  Table=admireDB.aerodata_asym_ext.CCDAAL.newTable  ExtrapMethod=Clip  InternalRulePriority=Speed  RndMeth=Simplest  InputSameDT=on
      settings: InputPortMap=u0,u1
  CCDAL_DE_ALFA : Lookup_n-D  BreakpointsForDimension1=admireDB.aerodata_asym_ext.CCDAL.breakpoints.ALFA  BreakpointsForDimension2=admireDB.aerodata_asym_ext.CCDAL.breakpoints.DE  BreakpointsForDimension3=[5, 7]  Table=admireDB.aerodata_asym_ext.CCDAL.newTable  ExtrapMethod=Clip  InternalRulePriority=Speed  RndMeth=Simplest  InputSameDT=on
      settings: InputPortMap=u0,u1
  CCDAL_DE_ALFA_1 : Lookup_n-D  BreakpointsForDimension1=admireDB.aerodata_asym_ext.CCDAL.breakpoints.ALFA  BreakpointsForDimension2=admireDB.aerodata_asym_ext.CCDAL.breakpoints.DE  BreakpointsForDimension3=[5, 7]  Table=admireDB.aerodata_asym_ext.CCDAL.newTable  ExtrapMethod=Clip  InternalRulePriority=Speed  RndMeth=Simplest  InputSameDT=on
      settings: InputPortMap=u0,u1
  CCEDAY_QA_M : Lookup_n-D  BreakpointsForDimension1=admireDB.aerodata_asym_ext.CCEDAY.breakpoints.M  BreakpointsForDimension2=admireDB.aerodata_asym_ext.CCEDAY.breakpoints.QA  BreakpointsForDimension3=[5, 7]  Table=admireDB.aerodata_asym_ext.CCEDAY.newTable  ExtrapMethod=Clip  InternalRulePriority=Speed  RndMeth=Simplest  InputSameDT=on
      settings: InputPortMap=u0,u1
  Degrees to Radians : simulink_extras/Transformations/Degrees to Radians
  Product : Product  Inputs=**
  Product1 : Product  Inputs=**
  Product2 : Product
  Product3 : Product
  Sign : Signum
  Sum : Sum  Inputs=|++
  Sum1 : Sum  Inputs=|++
  Sum2 : Sum  Inputs=|+-
  dE_cnst : Constant  Value=0.0
  Ccday : Outport
  wires:
  Sum2/1 -> Product1/2
  CCDAL_DE_ALFA_1/1 -> Sum2/2
  CCDAL_DE_ALFA/1 -> Sum2/1
  CCEDAY_QA_M/1 -> Product3/2
  Product2/1 -> Sum1/1
  Sum1/1 -> Ccday/1
  dAY/1 -> Abs/1, Degrees to Radians/1, Sign/1
  CCDAAL_DA_ALFA/1 -> Product/2
  Sign/1 -> Product/1
  Abs/1 -> CCDAAL_DA_ALFA/2
  Product/1 -> Sum/1
  dE_cnst/1 -> CCDAL_DE_ALFA_1/2
  dEY/1 -> CCDAL_DE_ALFA/2
  angleOfAttack_deg/1 -> CCDAL_DE_ALFA/1, CCDAL_DE_ALFA_1/1, CCDAAL_DA_ALFA/1
  Degrees to Radians/1 -> Product1/1, Product3/1
  Product1/1 -> Sum/2
  eoeff/1 -> Product2/2
  Sum/1 -> Product2/1
  mach_nd/1 -> CCEDAY_QA_M/1
  qacorr/1 -> CCEDAY_QA_M/2
  Product3/1 -> Sum1/2

== system aerotest/CentripetalForceCoefficient/MachRegion1/Ccdayb/Ccdayb_ ==
  angleOfAttack_deg : Inport
  dAY : Inport  Port=2
  angleOfSideslip_deg : Inport  Port=3
  eoeff : Inport  Port=4
  Abs : Abs
  Abs1 : Abs
  Abs2 : Abs
  CCDABAL_ALFA : Lookup_n-D  NumberOfTableDimensions=1  BreakpointsForDimension1=admireDB.aerodata_asym_ext.CCDABAL.breakpoints.ALFA  BreakpointsForDimension3=[5, 7]  Table=admireDB.aerodata_asym_ext.CCDABAL.newTable  ExtrapMethod=Clip  InternalRulePriority=Speed  RndMeth=Simplest  InputSameDT=on
  Constant : Constant  Value=30
  Constant1 : Constant  Value=20
  Product : Product  Inputs=**/*/*
  Ccdayb : Outport
  wires:
  eoeff/1 -> Product/6
  dAY/1 -> Abs/1
  angleOfAttack_deg/1 -> Abs2/1
  Product/1 -> Ccdayb/1
  CCDABAL_ALFA/1 -> Product/1
  Abs/1 -> Product/2
  Constant/1 -> Product/3
  angleOfSideslip_deg/1 -> Abs1/1
  Abs1/1 -> Product/4
  Constant1/1 -> Product/5
  Abs2/1 -> CCDABAL_ALFA/1

== system aerotest/CentripetalForceCoefficient/MachRegion1/Ccdna/Ccdna_ ==
  dNE : Inport
  angleOfAttack_deg : Inport  Port=2
  dNA : Inport  Port=3
  CCDNAAL_DNE_ALFA : Lookup_n-D  BreakpointsForDimension1=admireDB.aerodata_asym_ext.CCDNAAL.breakpoints.ALFA  BreakpointsForDimension2=admireDB.aerodata_asym_ext.CCDNAAL.breakpoints.DNE  BreakpointsForDimension3=[5, 7]  Table=admireDB.aerodata_asym_ext.CCDNAAL.newTable  ExtrapMethod=Clip  InternalRulePriority=Speed  RndMeth=Simplest  InputSameDT=on
      settings: InputPortMap=u0,u1
  Degrees to Radians : simulink_extras/Transformations/Degrees to Radians
  Product : Product
  Ccdna : Outport
  wires:
  Product/1 -> Ccdna/1
  Degrees to Radians/1 -> Product/2
  CCDNAAL_DNE_ALFA/1 -> Product/1
  dNA/1 -> Degrees to Radians/1
  dNE/1 -> CCDNAAL_DNE_ALFA/2
  angleOfAttack_deg/1 -> CCDNAAL_DNE_ALFA/1

== system aerotest/CentripetalForceCoefficient/MachRegion1/Ccdr/Ccdr_ ==
  angleOfAttack_deg : Inport
  dR : Inport  Port=2
  angleOfSideslip_deg : Inport  Port=3
  qacorr : Inport  Port=4
  mach_nd : Inport  Port=5
  Abs : Abs
  CCBDRAL_ALFA_DR_BETA : Lookup_n-D  NumberOfTableDimensions=3  BreakpointsForDimension1=admireDB.aerodata_asym_ext.CCBDRAL.breakpoints.ALFA  BreakpointsForDimension2=admireDB.aerodata_asym_ext.CCBDRAL.breakpoints.DR  BreakpointsForDimension3=admireDB.aerodata_asym_ext.CCBDRAL.breakpoints.BETA  Table=admireDB.aerodata_asym_ext.CCBDRAL.newTable  ExtrapMethod=Clip  InternalRulePriority=Speed  RndMeth=Simplest  InputSameDT=on
      settings: InputPortMap=u0,u1,u2
  CCEDR_QA_M : Lookup_n-D  BreakpointsForDimension1=admireDB.aerodata_asym_ext.CCEDR.breakpoints.M  BreakpointsForDimension2=admireDB.aerodata_asym_ext.CCEDR.breakpoints.QA  BreakpointsForDimension3=[5, 7]  Table=admireDB.aerodata_asym_ext.CCEDR.newTable  ExtrapMethod=Clip  InternalRulePriority=Speed  RndMeth=Simplest  InputSameDT=on
      settings: InputPortMap=u0,u1
  Product : Product  Inputs=**
  Ccdr : Outport
  wires:
  Abs/1 -> CCBDRAL_ALFA_DR_BETA/3
  angleOfAttack_deg/1 -> CCBDRAL_ALFA_DR_BETA/1
  Product/1 -> Ccdr/1
  CCEDR_QA_M/1 -> Product/2
  CCBDRAL_ALFA_DR_BETA/1 -> Product/1
  angleOfSideslip_deg/1 -> Abs/1
  dR/1 -> CCBDRAL_ALFA_DR_BETA/2
  qacorr/1 -> CCEDR_QA_M/2
  mach_nd/1 -> CCEDR_QA_M/1

== system aerotest/CentripetalForceCoefficient/MachRegion1/Ccp/Ccp_ ==
  angleOfAttack_deg : Inport
  pc : Inport  Port=2
  CCPAL_ALFA : Lookup_n-D  NumberOfTableDimensions=1  BreakpointsForDimension1=admireDB.aerodata_asym_ext.CCPAL.breakpoints.ALFA  BreakpointsForDimension3=[5, 7]  Table=admireDB.aerodata_asym_ext.CCPAL.newTable  ExtrapMethod=Clip  InternalRulePriority=Speed  RndMeth=Simplest  InputSameDT=on
  Product : Product
  Ccp : Outport
  wires:
  angleOfAttack_deg/1 -> CCPAL_ALFA/1
  CCPAL_ALFA/1 -> Product/1
  pc/1 -> Product/2
  Product/1 -> Ccp/1

== system aerotest/CentripetalForceCoefficient/MachRegion1/Ccpbeta/Ccpbeta_ ==
  angleOfSideslip_deg : Inport
  pc : Inport  Port=2
  angleOfAttack_deg : Inport  Port=3
  Abs : Abs
  CCPBA_BETA_ALFA : Lookup_n-D  BreakpointsForDimension1=admireDB.aerodata_asym_ext.CCPBA.breakpoints.ALFA  BreakpointsForDimension2=admireDB.aerodata_asym_ext.CCPBA.breakpoints.BETA  BreakpointsForDimension3=[5, 7]  Table=admireDB.aerodata_asym_ext.CCPBA.newTable  ExtrapMethod=Clip  InternalRulePriority=Speed  RndMeth=Simplest  InputSameDT=on
      settings: InputPortMap=u0,u1
  Product : Product
  Ccpbeta : Outport
  wires:
  Abs/1 -> CCPBA_BETA_ALFA/2
  angleOfSideslip_deg/1 -> Abs/1
  angleOfAttack_deg/1 -> CCPBA_BETA_ALFA/1
  Product/1 -> Ccpbeta/1
  pc/1 -> Product/2
  CCPBA_BETA_ALFA/1 -> Product/1

== system aerotest/CentripetalForceCoefficient/MachRegion1/Ccr/Ccr_ ==
  dN : Inport
  angleOfAttack_deg : Inport  Port=2
  rc : Inport  Port=3
  CCRAL_DNV_ALFA : Lookup_n-D  BreakpointsForDimension1=admireDB.aerodata_asym_ext.CCRAL.breakpoints.ALFA  BreakpointsForDimension2=admireDB.aerodata_asym_ext.CCRAL.breakpoints.DNV  BreakpointsForDimension3=[5, 7]  Table=admireDB.aerodata_asym_ext.CCRAL.newTable  ExtrapMethod=Clip  InternalRulePriority=Speed  RndMeth=Simplest  InputSameDT=on
      settings: InputPortMap=u0,u1
  Product : Product
  Ccr : Outport
  wires:
  CCRAL_DNV_ALFA/1 -> Product/1
  dN/1 -> CCRAL_DNV_ALFA/2
  angleOfAttack_deg/1 -> CCRAL_DNV_ALFA/1
  rc/1 -> Product/2
  Product/1 -> Ccr/1

== system aerotest/CentripetalForceCoefficient/MachRegion1/Ccrbeta/Ccrbeta_ ==
  angleOfSideslip_deg : Inport
  angleOfAttack_deg : Inport  Port=2
  rc : Inport  Port=3
  Abs : Abs
  Abs1 : Abs
  CCRBA_BETA_ALFA : Lookup_n-D  BreakpointsForDimension1=admireDB.aerodata_asym_ext.CCRBA.breakpoints.ALFA  BreakpointsForDimension2=admireDB.aerodata_asym_ext.CCRBA.breakpoints.BETA  BreakpointsForDimension3=[5, 7]  Table=admireDB.aerodata_asym_ext.CCRBA.newTable  ExtrapMethod=Clip  InternalRulePriority=Speed  RndMeth=Simplest  InputSameDT=on
      settings: InputPortMap=u0,u1
  Product : Product
  Ccrbeta : Outport
  wires:
  Abs1/1 -> CCRBA_BETA_ALFA/1
  Abs/1 -> CCRBA_BETA_ALFA/2
  angleOfSideslip_deg/1 -> Abs/1
  angleOfAttack_deg/1 -> Abs1/1
  Product/1 -> Ccrbeta/1
  rc/1 -> Product/2
  CCRBA_BETA_ALFA/1 -> Product/1

== system aerotest/CentripetalForceCoefficient/MachRegion2/Ccbcai/Ccbcai_ ==
  cai : Inport
  angleOfAttack_deg : Inport  Port=2
  angleOfSideslip_deg : Inport  Port=3
  CCBCAI_CAI_ALFA : Lookup_n-D  BreakpointsForDimension1=admireDB.aerodata_asym_ext.CCBCAI.breakpoints.ALFA  BreakpointsForDimension2=admireDB.aerodata_asym_ext.CCBCAI.breakpoints.CAI  BreakpointsForDimension3=[5, 7]  Table=admireDB.aerodata_asym_ext.CCBCAI.newTable  ExtrapMethod=Clip  InternalRulePriority=Speed  RndMeth=Simplest  InputSameDT=on
      settings: InputPortMap=u0,u1
  Degrees to Radians : simulink_extras/Transformations/Degrees to Radians
  Product : Product
  Ccbcai : Outport
  wires:
  Product/1 -> Ccbcai/1
  cai/1 -> CCBCAI_CAI_ALFA/2
  angleOfAttack_deg/1 -> CCBCAI_CAI_ALFA/1
  angleOfSideslip_deg/1 -> Degrees to Radians/1
  Degrees to Radians/1 -> Product/2
  CCBCAI_CAI_ALFA/1 -> Product/1

== system aerotest/CentripetalForceCoefficient/MachRegion2/Ccbde/Ccbde_ ==
  angleOfAttack_deg : Inport
  dEI : Inport  Port=2
  angleOfSideslip_deg : Inport  Port=3
  eieff : Inport  Port=4
  dEY : Inport  Port=5
  eoeff : Inport  Port=6
  Abs : Abs
  CCDEB_ALFA_DE_BETA : Lookup_n-D  NumberOfTableDimensions=3  BreakpointsForDimension1=admireDB.aerodata_asym_ext.CCDEB.breakpoints.ALFA  BreakpointsForDimension2=admireDB.aerodata_asym_ext.CCDEB.breakpoints.DE  BreakpointsForDimension3=admireDB.aerodata_asym_ext.CCDEB.breakpoints.BETA  Table=admireDB.aerodata_asym_ext.CCDEB.newTable  ExtrapMethod=Clip  InternalRulePriority=Speed  RndMeth=Simplest  InputSameDT=on
      settings: InputPortMap=u0,u1,u2
  CCDEB_ALFA_DE_BETA1 : Lookup_n-D  NumberOfTableDimensions=3  BreakpointsForDimension1=admireDB.aerodata_asym_ext.CCDEB.breakpoints.ALFA  BreakpointsForDimension2=admireDB.aerodata_asym_ext.CCDEB.breakpoints.DE  BreakpointsForDimension3=admireDB.aerodata_asym_ext.CCDEB.breakpoints.BETA  Table=admireDB.aerodata_asym_ext.CCDEB.newTable  ExtrapMethod=Clip  InternalRulePriority=Speed  RndMeth=Simplest  InputSameDT=on
      settings: InputPortMap=u0,u1,u2
  Product : Product
  Product1 : Product
  Product2 : Product
  Sign : Signum
  Sum : Sum  Inputs=|++
  Ccbde : Outport
  wires:
  Product2/1 -> Ccbde/1
  angleOfAttack_deg/1 -> CCDEB_ALFA_DE_BETA/1, CCDEB_ALFA_DE_BETA1/1
  dEI/1 -> CCDEB_ALFA_DE_BETA/2
  eieff/1 -> Product/2
  CCDEB_ALFA_DE_BETA/1 -> Product/1
  dEY/1 -> CCDEB_ALFA_DE_BETA1/2
  eoeff/1 -> Product1/2
  CCDEB_ALFA_DE_BETA1/1 -> Product1/1
  Product/1 -> Sum/1
  Product1/1 -> Sum/2
  Sum/1 -> Product2/1
  Sign/1 -> Product2/2
  angleOfSideslip_deg/1 -> Sign/1, Abs/1
  Abs/1 -> CCDEB_ALFA_DE_BETA/3, CCDEB_ALFA_DE_BETA1/3

== system aerotest/CentripetalForceCoefficient/MachRegion2/Ccbdle/Ccbdle_ ==
  angleOfAttack_deg : Inport
  angleOfSideslip_deg : Inport  Port=2
  dLE : Inport  Port=3
  tflow : Inport  Port=4
  tfhigh : Inport  Port=5
  Abs : Abs
  CCBDLE_M_ALFA : Lookup_n-D  BreakpointsForDimension1=admireDB.aerodata_asym_ext.CCBDLE.breakpoints.ALFA  BreakpointsForDimension2=admireDB.aerodata_asym_ext.CCBDLE.breakpoints.M  BreakpointsForDimension3=[5, 7]  Table=admireDB.aerodata_asym_ext.CCBDLE.newTable  ExtrapMethod=Clip  InternalRulePriority=Speed  RndMeth=Simplest  InputSameDT=on
      settings: InputPortMap=u0,u1
  CCDLEB_ALFA_BETA_DLE : Lookup_n-D  NumberOfTableDimensions=3  BreakpointsForDimension1=admireDB.aerodata_asym_ext.CCDLEB.breakpoints.ALFA  BreakpointsForDimension2=admireDB.aerodata_asym_ext.CCDLEB.breakpoints.BETA  BreakpointsForDimension3=admireDB.aerodata_asym_ext.CCDLEB.breakpoints.DLE  Table=admireDB.aerodata_asym_ext.CCDLEB.newTable  ExtrapMethod=Clip  InternalRulePriority=Speed  RndMeth=Simplest  InputSameDT=on
      settings: InputPortMap=u0,u1,u2
  Constant : Constant  Value=0.5
  Constant1 : Constant  Value=1/27
  Degrees to Radians : simulink_extras/Transformations/Degrees to Radians
  Product : Product  Inputs=3
  Product1 : Product  Inputs=5
  Sign : Signum
  Sum : Sum  Inputs=|++
  Ccbdle : Outport
  wires:
  Constant/1 -> CCBDLE_M_ALFA/2
  angleOfSideslip_deg/1 -> Degrees to Radians/1, Sign/1, Abs/1
  Abs/1 -> CCDLEB_ALFA_BETA_DLE/2
  tflow/1 -> Product/2
  CCDLEB_ALFA_BETA_DLE/1 -> Product/1
  Sign/1 -> Product/3
  Product/1 -> Sum/1
  angleOfAttack_deg/1 -> CCDLEB_ALFA_BETA_DLE/1, CCBDLE_M_ALFA/1
  Degrees to Radians/1 -> Product1/1
  CCBDLE_M_ALFA/1 -> Product1/4
  tfhigh/1 -> Product1/5
  Constant1/1 -> Product1/3
  dLE/1 -> CCDLEB_ALFA_BETA_DLE/3, Product1/2
  Product1/1 -> Sum/2
  Sum/1 -> Ccbdle/1

== system aerotest/CentripetalForceCoefficient/MachRegion2/Ccbdn/Ccbdn_ ==
  angleOfAttack_deg : Inport
  dN : Inport  Port=2
  angleOfSideslip_deg : Inport  Port=3
  Abs : Abs
  CCDNB_ALFA_DN_BETA : Lookup_n-D  NumberOfTableDimensions=3  BreakpointsForDimension1=admireDB.aerodata_asym_ext.CCDNB.breakpoints.ALFA  BreakpointsForDimension2=admireDB.aerodata_asym_ext.CCDNB.breakpoints.DN  BreakpointsForDimension3=admireDB.aerodata_asym_ext.CCDNB.breakpoints.BETA  Table=admireDB.aerodata_asym_ext.CCDNB.newTable  ExtrapMethod=Clip  InternalRulePriority=Speed  RndMeth=Simplest  InputSameDT=on
      settings: InputPortMap=u0,u1,u2
  Product : Product
  Sign : Signum
  Ccbdn : Outport
  wires:
  angleOfAttack_deg/1 -> CCDNB_ALFA_DN_BETA/1
  dN/1 -> CCDNB_ALFA_DN_BETA/2
  angleOfSideslip_deg/1 -> Sign/1, Abs/1
  Abs/1 -> CCDNB_ALFA_DN_BETA/3
  CCDNB_ALFA_DN_BETA/1 -> Product/1
  Sign/1 -> Product/2
  Product/1 -> Ccbdn/1
